simulink model "plantM"  (Simulink 7.4)
settings: Solver=ode45  StartTime=0.0  StopTime=10.0  RelTol=1e-3
values from neighbouring files (symbols this model uses):
  Ga = 3    [a2_data_input_examsim1.m]
  Gf = Gr/(Kd*Gs)    [a3_process_input.m]
  Gr = 1    [a2_data_input_examsim1.m]
  Gs = 1    [a2_data_input_examsim1.m]
  Kd = 2    [a2_data_input_examsim1.m]
undefined symbols (not defined in the file or in its folder): Gp_nominal_den, Gp_nominal_num, W1mod_den, W1mod_num, W2mod_den, W2mod_num
settings Model: Creator=Mauricio  LastModifiedBy=Vittorio

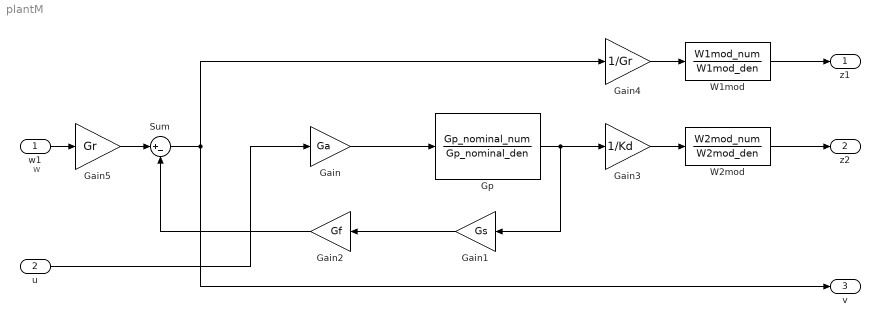
== system plantM ==
  note: w
  w1 : Inport  OutDataType=fixdt(1, 16)  OutScaling=2^0
  u : Inport  Port=2  OutDataType=fixdt(1, 16)  OutScaling=2^0
  Gain : Gain  Gain=Ga  ParameterDataType=fixdt(1, 16)  ParameterScaling=2^0  OutDataType=fixdt(1, 16)  OutScaling=2^0
  Gain1 : Gain  Gain=Gs  ParameterDataType=fixdt(1, 16)  ParameterScaling=2^0  OutDataType=fixdt(1, 16)  OutScaling=2^0
  Gain2 : Gain  Gain=Gf  ParameterDataType=fixdt(1, 16)  ParameterScaling=2^0  OutDataType=fixdt(1, 16)  OutScaling=2^0
  Gain3 : Gain  Gain=1/Kd  ParameterDataType=fixdt(1, 16)  ParameterScaling=2^0  OutDataType=fixdt(1, 16)  OutScaling=2^0
  Gain4 : Gain  Gain=1/Gr  ParameterDataType=fixdt(1, 16)  ParameterScaling=2^0  OutDataType=fixdt(1, 16)  OutScaling=2^0
  Gain5 : Gain  Gain=Gr  ParameterDataType=fixdt(1, 16)  ParameterScaling=2^0  OutDataType=fixdt(1, 16)  OutScaling=2^0
  Gp : TransferFcn  Numerator=Gp_nominal_num  Denominator=Gp_nominal_den
  Sum : Sum  Inputs=|+-  OutDataType=fixdt(1, 16)  OutScaling=2^0
  W1mod : TransferFcn  Numerator=W1mod_num  Denominator=W1mod_den
  W2mod : TransferFcn  Numerator=W2mod_num  Denominator=W2mod_den
  z1 : Outport  OutDataType=fixdt(1, 16)  OutScaling=2^0
  z2 : Outport  Port=2  OutDataType=fixdt(1, 16)  OutScaling=2^0
  v : Outport  Port=3  OutDataType=fixdt(1, 16)  OutScaling=2^0
  wires:
  Gp/1 -> Gain1/1, Gain3/1
  W1mod/1 -> z1/1
  W2mod/1 -> z2/1
  u/1 -> Gain/1
  w1/1 -> Gain5/1
  Sum/1 -> v/1, Gain4/1
  Gain/1 -> Gp/1
  Gain2/1 -> Sum/2
  Gain1/1 -> Gain2/1
  Gain3/1 -> W2mod/1
  Gain4/1 -> W1mod/1
  Gain5/1 -> Sum/1
